simulink model "Kinematics"  (R2017b)
settings: Solver=VariableStepAuto  StartTime=0.0  StopTime=10.0  RelTol=1e-3
settings Model: Creator=Kalana  LastModifiedBy=Kalana

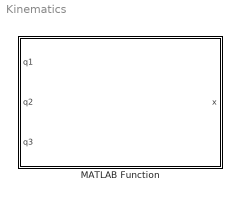
== system Kinematics ==
  MATLAB Function : MATLAB Function  TreatAsAtomicUnit=on

== matlab function Kinematics/MATLAB Function ==
  data: q1 input; x output; q2 input; q3 input
function x = Kinematics(q1, q2, q3)

leg = [0.265;
       0;
       0;
       1];
   
Trans0_3 = [cosd(q1)*cosd(q2-q3),   cosd(q1)*sind(q2-q3),   -sind(q1),      0.2*cosd(q1)*cosd(q2)+0.1225*cosd(q1)-0.0525*sind(q1);
            sind(q2-q3),            -cosd(q2-q3),           0,              0.2*sind(q2);
            -sind(q1)*cosd(q2-q3),  -sind(q1)*sind(q2-q3),  -cosd(q1),      -0.2*sind(q1)*cosd(q2)-0.1225*sind(q1)-0.0525*cosd(q1);
            0,                      0,                      0,              1];
        
x_temp = Trans0_3*leg;

x = x_temp(1:3);
